simulink model "ev"  (R2021a)
settings: Solver=ode4  StartTime=0  StopTime=1082  FixedStep=sim_dt  RelTol=1e-3
model workspace (MAT data in the model file):
  T_eff_bp = [-270; -210; -150; -90; -30; 30; 90; 150; 210; 270]
  T_eff_bp_2 = [-270; -210; -150; -90; -30; 30; 90; 150; 210; 270]
  losses_table = [108927.107777  108927.107777  108927.107777  108927.107777  108927.107777  108927.107777  108927.107777  108927.107777  108927.107777  108927.107777; 7820.2782368  7820.2782368  7820.2782368  7820.2782368  7820.2782368  7820.2782368  7820.2782368  7820.2782368  7820.2782368  7820.2782368; 7820.17609997  7820.17609997  7820.17609997  7820.17609997  7820.17609997  7820.17609997  7820.17609997  7820.17609997  7820.17609997  7820.17609997; 7820.2782368  7820.2782368  7820.2782368  7820.2782368  7820.2782368  7820.2782368  7820.2782368  7820.2782368  7820.2782368  7820.2782368; 7820.2782368  7820.2782368  7820.2782368  7820.2782368  7820.2782368  7820.2782368  7820.2782368  7820.2782368  7820.2782368  7820.2782368; 7820.2782368  7820.2782368  7820.2782368  7820.2782368  7820.2782368  7820.2782368  7820.2782368  7820.2782368  7820.2782368  7820.2782368; 7820.2782368  7820.2782368  7820.2782368  7820.2782368  7820.2782368  7820.2782368  7820.2782368  7820.2782368  7820.2782368  7820.2782368; 7820.26172359  7820.26172359  7820.26172359  7820.26172359  7820.26172359  7820.26172359  7820.26172359  7820.26172359  7820.26172359  7820.26172359; 7820.2782368  7820.2782368  7820.2782368  7820.2782368  7820.2782368  7820.2782368  7820.2782368  7820.2782368  7820.2782368  7820.2782368; 9345.38006027  9345.38006027  9345.38006027  9345.38006027  9345.38006027  9345.38006027  9345.38006027  9345.38006027  9345.38006027  9345.38006027]
  losses_table_2 = [108927.107777  108927.107777  108927.107777  108927.107777  108927.107777  108927.107777  108927.107777  108927.107777  108927.107777  108927.107777; 7820.2782368  7820.2782368  7820.2782368  7820.2782368  7820.2782368  7820.2782368  7820.2782368  7820.2782368  7820.2782368  7820.2782368; 7820.17609997  7820.17609997  7820.17609997  7820.17609997  7820.17609997  7820.17609997  7820.17609997  7820.17609997  7820.17609997  7820.17609997; 7820.2782368  7820.2782368  7820.2782368  7820.2782368  7820.2782368  7820.2782368  7820.2782368  7820.2782368  7820.2782368  7820.2782368; 7820.2782368  7820.2782368  7820.2782368  7820.2782368  7820.2782368  7820.2782368  7820.2782368  7820.2782368  7820.2782368  7820.2782368; 7820.2782368  7820.2782368  7820.2782368  7820.2782368  7820.2782368  7820.2782368  7820.2782368  7820.2782368  7820.2782368  7820.2782368; 7820.2782368  7820.2782368  7820.2782368  7820.2782368  7820.2782368  7820.2782368  7820.2782368  7820.2782368  7820.2782368  7820.2782368; 7820.26172359  7820.26172359  7820.26172359  7820.26172359  7820.26172359  7820.26172359  7820.26172359  7820.26172359  7820.26172359  7820.26172359; 7820.2782368  7820.2782368  7820.2782368  7820.2782368  7820.2782368  7820.2782368  7820.2782368  7820.2782368  7820.2782368  7820.2782368; 9345.38006027  9345.38006027  9345.38006027  9345.38006027  9345.38006027  9345.38006027  9345.38006027  9345.38006027  9345.38006027  9345.38006027]
  w_eff_bp = [0; 888.888888889; 1777.77777778; 2666.66666667; 3555.55555556; 4444.44444444; 5333.33333333; 6222.22222222; 7111.11111111; 8000]
  w_eff_bp_2 = [0; 888.888888889; 1777.77777778; 2666.66666667; 3555.55555556; 4444.44444444; 5333.33333333; 6222.22222222; 7111.11111111; 8000]
undefined symbols (not defined in the file): Af, alpha, Bt, C, C_fa, C_free, C_sa_bat, C_sa_uc, Cd, Cmax, Continuous, Crr, DoD, effi, etaFD, etaG, FD, G, gear, Iucmax, m, M1m, M2m, Max, npar, npar_free, npara, nparf, nparfa, nparsa_bat, nparsa_UC, nser, nser_free, nserfa, nsersa_bat, nsersa_UC, Qbat, regenmax, Ri_BP, RL, ro, Rsc, Rsc_A, Rsc_F, Rsc_sa_bat, Rsc_sa_uc, rw, sim_dt, SOC_BP, SoCbatmax, SoCbatmin, SoCucmax, SoCucmin, speed, torque, VinBat, Voc_BP, Vuc, Vuc_fa, Vuc_free ... (+2)
libraries: autolibshared x41, simulink x26, autolibdcdc x13, autolibdatasheetbattery x7, autolibmappedmotor x6, fl_lib x3, nesl_utility x3, spsSupercapacitorLib x3, pid_lib x1
(part 1 of 18)
settings Model: OrderedModelArguments=off  Creator=GIT5SLP  LastModifiedBy=gzdan
settings DataIOCC: ReturnWorkspaceOutputs=off
settings DebuggingCC: SFMachineParentedDataDiag=warning  ArithmeticOperatorsInVariantConditions=warning
settings SFSimCC: SimUseLocalCustomCode=off  CustomCodeUndefinedFunction=UseInterfaceOnly
settings RTWCC: RTWUseLocalCustomCode=off
settings CodeAppCC: StateflowObjectComments=on

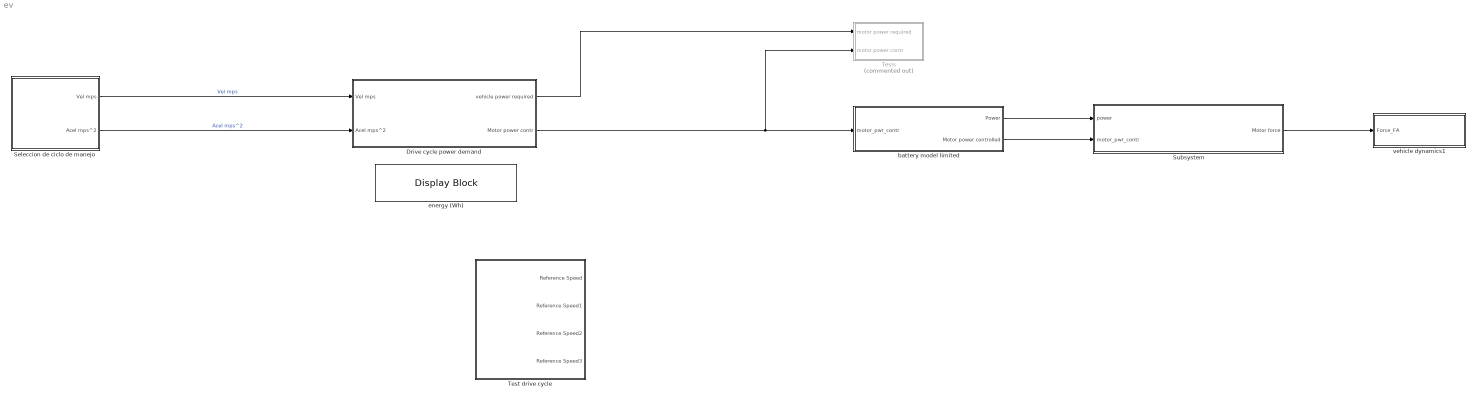
== system ev ==
  Drive cycle power demand : Subsystem
  Seleccion de ciclo de manejo : Subsystem
  Subsystem : Subsystem
  Tesis : Subsystem  Commented=on
  Test drive cycle : Subsystem
  battery model limited : Subsystem
  "energy (Wh) " : DisplayBlock  LabelPosition=Hide  Format=shortEng  Transparency=1
  vehicle dynamics1 : Subsystem
  wires:
  Subsystem/1(Motor force) -> vehicle dynamics1/1("Force_FA ")
  battery model limited/2(Motor power controlled) -> Subsystem/2(motor_pwr_contr)
  battery model limited/1(Power) -> Subsystem/1(power)
  Drive cycle power demand/2(Motor power contr) -> Tesis/2(motor power contr), battery model limited/1(motor_pwr_contr)
  Seleccion de ciclo de manejo/1(Vel mps) -> Drive cycle power demand/1(Vel mps)  "Vel mps"
  Seleccion de ciclo de manejo/2(Acel mps^2) -> Drive cycle power demand/2(Acel mps^2)  "Acel mps^2"
  Drive cycle power demand/1(vehicle power required) -> Tesis/1(motor power required)

== system ev/Drive cycle power demand ==
  Vel mps : Inport
  Acel mps^2 : Inport  Port=2
  Controller. Actual motor torque : Subsystem
  Gain : Gain  Gain=1/3600
  Integrator : Integrator
  Motor torque estimation : Subsystem
  Power estimation : Subsystem
  Scope : Scope
  Scope2 : Scope  NumInputPorts=2
  Scope3 : Scope
  Scope4 : Scope
  To Workspace : ToWorkspace  VariableName=veh_ener  SaveFormat=Structure With Time  SampleTime=-1
  Veh force estimation : Subsystem
  motor speed estimation : Subsystem
  vehicle power required : Outport
  Motor power contr : Outport  Port=2
  tag scope: vel_or=global
  wires:
  Acel mps^2/1 -> Veh force estimation/2(Acceleration)
  Controller. Actual motor torque/1(Motor power contr) -> Motor power contr/1, Scope2/2, Integrator/1
  Vel mps/1 -> motor speed estimation/1(vel_m/s), [vel_or], Scope/1, Power estimation/1(vel_m/s), Scope4/1, Veh force estimation/1(vel_m/s)
  Gain/1 -> To Workspace/1, Scope3/1
  Veh force estimation/1(Total force) -> Motor torque estimation/1(Force), Power estimation/2(Force)
  Power estimation/1(Power_motor_out) -> Scope2/1, vehicle power required/1, Controller. Actual motor torque/3(Power_motor_out)  "vehicle power required"
  Integrator/1 -> Gain/1
  Motor torque estimation/1(wheel torque) -> Controller. Actual motor torque/2(wheel torque)  "motor torque required"
  motor speed estimation/1(motor angular speed rad/s) -> Controller. Actual motor torque/1(motor angular speed)  "motor angular speed required"

== system ev/Seleccion de ciclo de manejo ==
  Constant : Constant  Value=0
  Constant1 : Constant
  Constant2 : Constant  Value=0
  Constant3 : Constant  Value=30*1.609344
  Drive Cycle Source : autolibshared/Drive Cycle Source  cycleVar=Artemis Rural Road  fileVar=cycleFTP75.mat  tfinal="1082  seconds, Cyclic"  cycleRepeat=on  outAccPort=on  outGearPort=off  gearList=No gear data  t_wot1=5  xdot_woto=0  xdot_wot1=30  t_wot2=20  xdot_wot2=0  t_wotend=30  srcUnit=m/s  outUnit=km/h  srcAccUnit=m/s/s  outAccUnit=m/s^2  dt=0  aMode=1  faultOption=off  velBnd=2  velBndUnit=mph  inUnit=m/s  timeBnd=1  failOption=off  stopSim=off  maxFaultCnt=10  maxFaultTime=2  maxTotFaultTime=15  traceOption=off  dtTrace=1  traceWindow=10  lastDCname=Artemis Rural Road  lastOutUnit=mph  lastDT=0  lastTB=1  lastSB=2  forceCalcBound=off
      settings: SourceProductBaseCode=PW,DR,MT,UV,VE
  Manual Switch : ManualSwitch
  Manual Switch1 : ManualSwitch  CurrentSetting=0
  Ramp : simulink/Sources/Ramp  slope=(30*1.609344)/400  start=0  InitialOutput=0
  Saturation Dynamic : simulink/Discontinuities/Saturation Dynamic  OutMin=[]  OutMax=[]  OutDataTypeStr=Inherit: Same as second input  OutDataType=fixdt(1, 16)  OutScaling=2^-10  DoSatur=off
  Scope1 : Scope  NumInputPorts=2
  Scope5 : Scope
  Subsystem : Subsystem
  Switch : Switch  Criteria=u2 ~= 0
  Switch1 : Switch  Criteria=u2 ~= 0
  Switch2 : Switch  Threshold=30*1.609344
  To Workspace7 : ToWorkspace  VariableName=vel_dc  SaveFormat=Structure With Time  SampleTime=-1
  Velocity : Subsystem
  Velocity1 : Subsystem
  degree : Constant  Value=0
  degree1 : Constant  Value=8
  Vel mps : Outport
  Acel mps^2 : Outport  Port=2
  tag scope: deg=global, switch=global
  wires:
  Constant1/1 -> Manual Switch/1
  Velocity1/1(Vel_m/s) -> Subsystem/1(Vel_m/s)  "vel_m/s"
  degree/1 -> Switch2/3, Manual Switch1/2
  Switch2/1 -> Manual Switch1/1
  Constant/1 -> Subsystem/2(Acel @vel const), Saturation Dynamic/3
  Switch1/1 -> Acel mps^2/1  "Acel mps^2"
  Subsystem/2(Accel) -> Switch1/3
  Constant2/1 -> Manual Switch/2
  Switch/1 -> Vel mps/1  "Vel mps"
  degree1/1 -> Switch2/1
  Saturation Dynamic/1 -> Velocity1/1(vel_km/h), Switch2/2, Scope1/1
  Ramp/1 -> Scope1/2, Saturation Dynamic/2
  Velocity/1(Vel_m/s) -> Switch/1  "vel_m/s"
  Manual Switch1/1 -> Scope5/1, [deg]
  Drive Cycle Source/2 -> Switch1/1
  Manual Switch/1 -> Switch1/2, [switch], Switch/2
  Drive Cycle Source/1 -> Velocity/1(vel_km/h), To Workspace7/1
  Constant3/1 -> Saturation Dynamic/1
  Subsystem/1(Vel) -> Switch/3

== system ev/Subsystem ==
  power : Inport
  motor_pwr_contr : Inport  Port=2
  1-D Lookup Table : Lookup_n-D  NumberOfTableDimensions=1  BreakpointsForDimension1=Continuous(:,1)  Table=Continuous(:,2)  InternalRulePriority=Speed  RndMeth=Simplest  InputSameDT=on
  1-D Lookup Table2 : Lookup_n-D  NumberOfTableDimensions=1  BreakpointsForDimension1=Continuous(:,1)  Table=-Continuous(:,2)  InternalRulePriority=Speed  RndMeth=Simplest  InputSameDT=on
  Constant : Constant  Value=0
  Constant1 : Constant
  Divide1 : Product  Inputs=**
  Divide2 : Product  Inputs=**
  Divide3 : Product  Inputs=*/
  Gain2 : Gain  Gain=30/pi
  Gain4 : Gain  Gain=0.95
  Gain5 : Gain  Gain=1/rw
  Gain6 : Gain  Gain=1/0.95
  Manual Switch : ManualSwitch  CurrentSetting=0
  Saturation Dynamic : simulink/Discontinuities/Saturation Dynamic  OutMin=[]  OutMax=[]  OutDataTypeStr=Inherit: Same as second input  OutDataType=fixdt(1, 16)  OutScaling=2^-10  DoSatur=off
  Scope : Scope
  Scope1 : Scope
  Switch : Switch  Criteria=u2 ~= 0
  Switch1 : Switch
  Switch2 : Switch  Criteria=u2 ~= 0
  motor speed estimation : Subsystem
  Motor force : Outport
  wires:
  motor_pwr_contr/1 -> Switch1/2
  Gain4/1 -> Divide1/1  "breaking torque"
  [gear_ratio] -> Divide1/2
  Divide1/1 -> Switch1/1
  Switch1/1 -> Gain5/1  "motor torque"
  Gain5/1 -> Motor force/1  "FORCE"
  [gear_ratio] -> Divide2/2
  Gain6/1 -> Divide2/1  "motor_torque"
  Divide2/1 -> Switch1/3
  Divide3/1 -> Switch/1, Scope/1  "torque"
  power/1 -> Divide3/1  "power"
  Gain2/1 -> 1-D Lookup Table2/1, 1-D Lookup Table/1
  1-D Lookup Table/1 -> Saturation Dynamic/1
  1-D Lookup Table2/1 -> Saturation Dynamic/3
  Saturation Dynamic/1 -> Gain4/1, Gain6/1
  Switch/1 -> Saturation Dynamic/2
  Constant/1 -> Switch/3
  motor speed estimation/1(motor angular speed) -> Manual Switch/2  "motor angular speed required"
  Manual Switch/1 -> Scope1/1, Gain2/1, Switch2/1, Switch2/2, Switch/2
  [mtr_speed] -> Manual Switch/1
  [Veh_real_bat2] -> motor speed estimation/1(vel_m/s)
  Switch2/1 -> Divide3/2
  Constant1/1 -> Switch2/3

== system ev/Tesis ==
  motor power required : Inport
  motor power contr : Inport  Port=2
  Battery model : Subsystem  Commented=on
  HESS : Subsystem
  battery model limitedmod : Subsystem  Commented=on
  wires:
  motor power contr/1 -> Battery model/1(motor_pwr_contr), battery model limitedmod/1(motor_pwr_contr), HESS/2(motor power contr)
  motor power required/1 -> HESS/1(motor power required)

== system ev/Test drive cycle ==
  Bus Selector{1..4} (4 alike) : BusSelector  OutputSignals=Fault.FaultCnt,Fault.CumFaultTime,Fault.Fault
  Drive Cycle Source{1..4} (4 alike) : autolibshared/Drive Cycle Source  cycleVar=Artemis Motorway 150 kmph  fileVar=cycleFTP75.mat  tfinal="1068  seconds, Cyclic"  cycleRepeat=on  outAccPort=off  outGearPort=off  gearList=No gear data  t_wot1=5  xdot_woto=0  xdot_wot1=30  t_wot2=20  xdot_wot2=0  t_wotend=30  srcUnit=m/s  outUnit=km/h  srcAccUnit=m/s/s  outAccUnit=m/s^2  dt=0  aMode=1  faultOption=on  velBnd=2  velBndUnit=mph  inUnit=m/s  timeBnd=1  failOption=on  stopSim=off  maxFaultCnt=100  maxFaultTime=200  maxTotFaultTime=1500  traceOption=off  dtTrace=1  traceWindow=10  lastDCname=Artemis Motorway 150 kmph  lastOutUnit=mph  lastDT=0  lastTB=1  lastSB=2  forceCalcBound=off
      settings: SourceProductBaseCode=PW,DR,MT,UV,VE
  Gain{1..4} (4 alike) : Gain  Gain=1/3.6
  Integrator{1..4} (4 alike) : Integrator
  Mux : Mux
  Mux1 : Mux
  Mux2 : Mux
  Scope{6..14} (9 alike) : Scope
  To Workspace1 : ToWorkspace  VariableName=zz_vel_fail  SaveFormat=Structure With Time  SampleTime=-1
  To Workspace2 : ToWorkspace  VariableName=zz_vel_fail_time  SaveFormat=Structure With Time  SampleTime=-1
  To Workspace3 : ToWorkspace  VariableName=zz_dist  SaveFormat=Structure With Time  SampleTime=-1
  Reference Speed : Outport
  Reference Speed1 : Outport  Port=2
  Reference Speed2 : Outport  Port=3
  Reference Speed3 : Outport  Port=4
  wires:
  Bus Selector2/1 -> Scope6/1  "<FaultCnt>"
  Bus Selector3/2 -> Scope11/1, Mux1/3  "<CumFaultTime>"
  [Vel_uc] -> Gain3/1, Drive Cycle Source3/1
  Bus Selector1/1 -> Scope8/1  "<FaultCnt>"
  Mux/1 -> To Workspace1/1
  Mux1/1 -> To Workspace2/1
  [Vel_act] -> Gain1/1, Drive Cycle Source1/1
  Drive Cycle Source3/1 -> Bus Selector3/1
  Bus Selector1/2 -> Mux1/2, Scope9/1  "<CumFaultTime>"
  Integrator3/1 -> Mux2/3
  Bus Selector4/2 -> Mux1/4, Scope13/1  "<CumFaultTime>"
  Drive Cycle Source1/1 -> Bus Selector2/1
  Drive Cycle Source4/1 -> Bus Selector4/1
  Bus Selector2/2 -> Mux1/1, Scope7/1  "<CumFaultTime>"
  Bus Selector4/3 -> Mux/4  "<Fault>"
  Bus Selector4/1 -> Scope12/1  "<FaultCnt>"
  [Vel_bat] -> Gain2/1, Drive Cycle Source2/1
  Bus Selector1/3 -> Mux/2  "<Fault>"
  Gain3/1 -> Integrator3/1
  Bus Selector3/3 -> Mux/3  "<Fault>"
  Bus Selector3/1 -> Scope10/1  "<FaultCnt>"
  Drive Cycle Source1/2 -> Reference Speed/1
  Mux2/1 -> Scope14/1, To Workspace3/1
  Gain1/1 -> Integrator1/1
  Drive Cycle Source2/1 -> Bus Selector1/1
  Integrator2/1 -> Mux2/2
  Gain4/1 -> Integrator4/1
  [Vel_pass] -> Gain4/1, Drive Cycle Source4/1
  Drive Cycle Source3/2 -> Reference Speed2/1
  Drive Cycle Source4/2 -> Reference Speed3/1
  Gain2/1 -> Integrator2/1
  Bus Selector2/3 -> Mux/1  "<Fault>"
  Integrator1/1 -> Mux2/1
  Integrator4/1 -> Mux2/4
  Drive Cycle Source2/2 -> Reference Speed1/1

== system ev/battery model limited ==
  motor_pwr_contr : Inport
  Gain : Gain  Gain=nser
  Gain1 : Gain  Gain=nser/npar
  Gain11 : Gain  Gain=(Qbat*VinBat*nser*npar)
  Gain2 : Gain  Gain=1/(Qbat*VinBat*nser*npar*3600)
  Gain3 : Gain  Gain=-1
  Ibatt1 : Scope
  Integrator2 : Integrator
  MATLAB Function : MATLAB Function  TreatAsAtomicUnit=on
  MATLAB Function2 : MATLAB Function  TreatAsAtomicUnit=on
  Mux13 : Mux  Inputs=3
  Mux14 : Mux  Inputs=3
  OCV : Lookup_n-D  NumberOfTableDimensions=1  BreakpointsForDimension1=SOC_BP  Table=Voc_BP  InternalRulePriority=Speed  RndMeth=Simplest  InputSameDT=on
  PMG_max : Lookup_n-D  NumberOfTableDimensions=1  BreakpointsForDimension1=SOC_BP  Table=Voc_BP*nser*1*50*npar  InternalRulePriority=Speed  RndMeth=Simplest  InputSameDT=on
  PMG_min : Lookup_n-D  NumberOfTableDimensions=1  BreakpointsForDimension1=SOC_BP  Table=-Voc_BP*nser*1*50*npar  InternalRulePriority=Speed  RndMeth=Simplest  InputSameDT=on
  Polim : Scope
  Pow1 : Scope
  Product : Product
  Product1 : Product
  Ri : Lookup_n-D  NumberOfTableDimensions=1  BreakpointsForDimension1=SOC_BP  Table=Ri_BP  InternalRulePriority=Speed  RndMeth=Simplest  InputSameDT=on
  Ri4 : Lookup_n-D  NumberOfTableDimensions=1  BreakpointsForDimension1=SOC_BP  Table=Ri_BP  InternalRulePriority=Speed  RndMeth=Simplest  InputSameDT=on
  SOC : Integrator  InitialCondition=(1-DoD)
  Saturation Dynamic : simulink/Discontinuities/Saturation Dynamic  OutMin=[]  OutMax=[]  OutDataTypeStr=Inherit: Same as second input  OutDataType=fixdt(1, 16)  OutScaling=2^-10  DoSatur=off
  Scope42 : Scope
  Scope43 : Scope
  Scope45 : Scope
  SoC : Scope  NumInputPorts=3
  Subtract : Sum  Inputs=+-
  Switch13 : Switch  Criteria=u2 > Threshold
  Vo : Scope
  Voc : Scope
  ener Wh : Scope
  iR : Scope
  iRt : Scope
  Power : Outport
  Motor power controlled : Outport  Port=2
  wires:
  Mux13/1 -> Scope42/1
  PMG_min/1 -> Saturation Dynamic/3, Scope43/1, Mux13/3
  Switch13/1 -> Gain1/1, iR/1
  Gain/1 -> MATLAB Function/1(OCV), Product/1, Subtract/1, Mux14/2, Voc/1  "OCV"
  Gain11/1 -> ener Wh/1
  Gain2/1 -> Integrator2/1, SOC/1
  motor_pwr_contr/1 -> Saturation Dynamic/2, Switch13/2, Mux13/1, Motor power controlled/1, MATLAB Function2/3(Pmot)
  Saturation Dynamic/1 -> Polim/1, MATLAB Function/3(P)
  Gain1/1 -> MATLAB Function2/1(Ri), Product1/2, MATLAB Function/2(Ri), iRt/1
  Ri/1 -> Switch13/1
  Ri4/1 -> Switch13/3
  MATLAB Function/1(I_batt) -> Ibatt1/1, Product1/1, MATLAB Function2/2(Ib), Product/2
  OCV/1 -> Vo/1, Gain/1
  Mux14/1 -> Scope45/1
  SOC/1 -> PMG_max/1, PMG_min/1, OCV/1, Ri/1, Ri4/1, SoC/1  "SOC"
  PMG_max/1 -> Saturation Dynamic/1, Mux13/2
  Integrator2/1 -> Gain11/1
  MATLAB Function2/1(Vb) -> Mux14/1  "Vb"
  Product/1 -> Pow1/1, Gain3/1, Gain2/1
  Gain3/1 -> Power/1
  [block] -> SoC/2
  Product1/1 -> Subtract/2
  Subtract/1 -> Mux14/3
  [modi] -> SoC/3
